simulink model "valid"  (R2020b)
settings: Solver=VariableStepAuto  StartTime=0.0  StopTime=10.0  RelTol=1e-3
undefined symbols (not defined in the file or in its folder): A, B, bm1, bm2, bp0, bp1, C, D, g, Jm, Jp, kaphi, ku1, ku2, ku3, ku4, l, La, m, Ra
libraries: simulink_extras x2
settings Model: Creator=Erick  LastModifiedBy=Erick

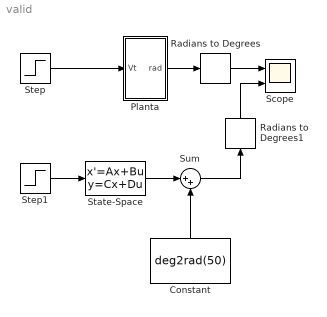
== system valid ==
  Constant : Constant  Value=deg2rad(50)
  Planta : Subsystem
  Radians to Degrees : simulink_extras/Transformations/Radians to Degrees
  Radians to Degrees1 : simulink_extras/Transformations/Radians to Degrees
  Scope : Scope  NumInputPorts=2
  State-Space : StateSpace  A=A  B=B  C=C  D=D  InitialCondition=0
  Step : Step  Time=5  Before=8.429  After=9.0  SampleTime=0
  Step1 : Step  Time=5  After=9-8.429  SampleTime=0
  Sum : Sum  Inputs=|++
  wires:
  Step/1 -> Planta/1(Vt)
  State-Space/1 -> Sum/1
  Step1/1 -> State-Space/1
  Constant/1 -> Sum/2
  Radians to Degrees/1 -> Scope/1
  Sum/1 -> Radians to Degrees1/1
  Radians to Degrees1/1 -> Scope/2
  Planta/1(rad) -> Radians to Degrees/1

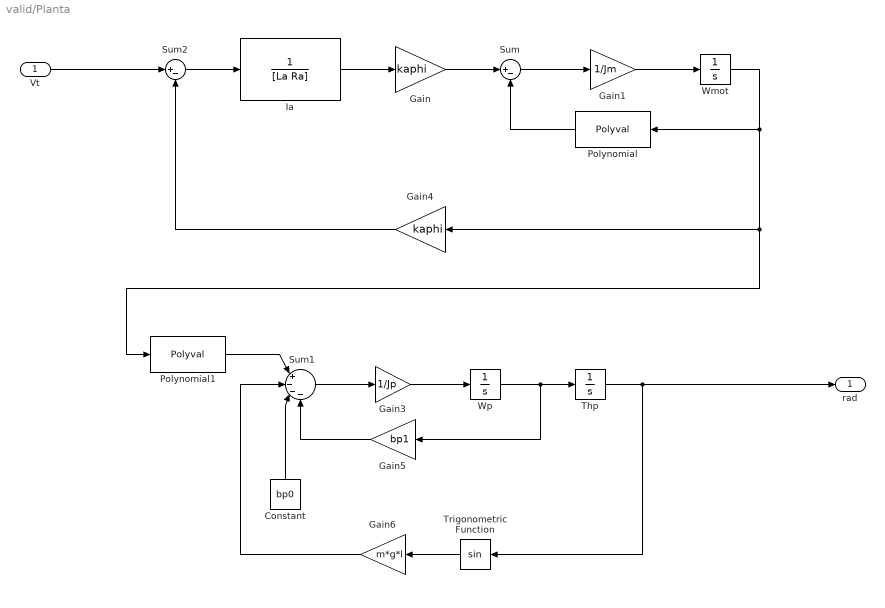
== system valid/Planta ==
  Vt : Inport
  Constant : Constant  Value=bp0
  Gain : Gain  Gain=kaphi
  Gain1 : Gain  Gain=1/Jm
  Gain3 : Gain  Gain=1/Jp
  Gain4 : Gain  Gain=kaphi
  Gain5 : Gain  Gain=bp1
  Gain6 : Gain  Gain=m*g*l
  Ia : TransferFcn  Denominator=[La Ra]
  Polynomial : Polyval  Coefs=[bm2, bm1, 0]
  Polynomial1 : Polyval  Coefs=[ku4, ku3, ku2, ku1, 0]
  Sum : Sum  Inputs=|+-
  Sum1 : Sum  Inputs=|+---
  Sum2 : Sum  Inputs=|+-
  Thp : Integrator  LimitOutput=on  UpperSaturationLimit=deg2rad(90)  LowerSaturationLimit=0
  Trigonometric Function : Trigonometry
  Wmot : Integrator
  Wp : Integrator
  rad : Outport
  wires:
  Sum2/1 -> Ia/1
  Sum/1 -> Gain1/1
  Wmot/1 -> Polynomial1/1, Gain4/1, Polynomial/1
  Trigonometric Function/1 -> Gain6/1
  Thp/1 -> rad/1, Trigonometric Function/1
  Gain1/1 -> Wmot/1
  Polynomial1/1 -> Sum1/1
  Gain6/1 -> Sum1/2
  Ia/1 -> Gain/1
  Gain3/1 -> Wp/1
  Gain/1 -> Sum/1
  Sum1/1 -> Gain3/1
  Constant/1 -> Sum1/3
  Vt/1 -> Sum2/1
  Gain5/1 -> Sum1/4
  Wp/1 -> Gain5/1, Thp/1
  Polynomial/1 -> Sum/2
  Gain4/1 -> Sum2/2
